simulink model "SPENCER_IK"  (R2023a)
settings: Solver=VariableStepAuto  StartTime=0.0  StopTime=10.0  RelTol=1e-3
model workspace (MAT data in the model file):
  C0 = [0.5 0.25 1]
  P = [1.14564392374 1.14333737187 1.13642700394 1.12494064556 1.10892454825 1.08844320316 1.06357908145 1.03443230217 1.0011202291 0.963776998212 0.922552977508 0.877614161573 ... (300 elements, 100x3)]
  P1 = [0 0 0]
  P5 = [1 0.5 2]
  P6 = [2 2 3]
  P8 = [0 0 1]
  R = 1.14564392374
  X = [0 0.0231772421242 0.0460988496987 0.0685120077079 0.0901695091058 0.110832481399 0.130273021303 0.148276708411 0.164644970158 0.179197271982 0.191773108544 0.202233774026 ... (300 elements, 300x1)]
  Y = [-0.220995 -0.219776262304 -0.216133491346 -0.210106865249 -0.201762854987 -0.191193491238 -0.178515349328 -0.163868263455 -0.147413784385 -0.129333397617 -0.109826521681 -0.0891083086369 ... (300 elements, 300x1)]
  Z = [0 0.00332775919732 0.00665551839465 0.00998327759197 0.0133110367893 0.0166387959866 0.0199665551839 0.0232943143813 0.0266220735786 0.0299498327759 0.0332775919732 0.0366053511706 ... (300 elements, 300x1)]
  a = 0.029995
  alpha = [0; 0.0634665182543; 0.126933036509; 0.190399554763; 0.253866073017; 0.317332591272; 0.380799109526; 0.44426562778; 0.507732146035; 0.571198664289; 0.634665182543; 0.698131700798; 0.761598219052; 0.825064737306; 0.888531255561; 0.951997773815; 1.01546429207; 1.07893081032; 1.14239732858; 1.20586384683; 1.26933036509; 1.33279688334; 1.3962634016; 1.45972991985; 1.5231964381; 1.58666295636; 1.65012947461; 1.71359599287; 1.77706251112; 1.84052902938; 1.90399554763; 1.96746206588; 2.03092858414; 2.09439510239; 2.15786162065; 2.2213281389; 2.28479465716; 2.34826117541; 2.41172769366; 2.47519421192; 2.53866073017; 2.60212724843; 2.66559376668; 2.72906028494; 2.79252680319; 2.85599332145; 2.9194598397; 2.98292635795; 3.04639287621; 3.10985939446; 3.17332591272; 3.23679243097; 3.30025894923; 3.36372546748; 3.42719198573; 3.49065850399; 3.55412502224; 3.6175915405; 3.68105805875; 3.74452457701; 3.80799109526; 3.87145761351; 3.93492413177; 3.99839065002; 4.06185716828; 4.12532368653; 4.18879020479; 4.25225672304; 4.3157232413; 4.37918975955; 4.4426562778; 4.50612279606; 4.56958931431; 4.63305583257; 4.69652235082; 4.75998886908; 4.82345538733; 4.88692190558; 4.95038842384; 5.01385494209; 5.07732146035; 5.1407879786; 5.20425449686; 5.26772101511; 5.33118753336; 5.39465405162; 5.45812056987; 5.52158708813; 5.58505360638; 5.64852012464; 5.71198664289; 5.77545316114; 5.8389196794; 5.90238619765; 5.96585271591; 6.02931923416; 6.09278575242; 6.15625227067; 6.21971878893; 6.28318530718]
  b = 0.191
  del = 0.16432586948
  dp = [-6 3]
  h : matlab.ui.Figure (value not decoded)
  n = 5
  nPt = 100
  nturns = 3
  out = Simulink.SimulationOutput
  out.Data.tout = [0 4.01901829042e-10 2.41141097425e-09 1.24589567003e-08 6.26966853305e-08 3.13885328481e-07 1.56982854424e-06 7.84954462301e-06 3.92481250169e-05 0.000196241026986 0.00063098304072 0.00113846260576 ... (4325 elements, 4325x1)]
  out.Metadata = Simulink.SimulationMetadata
  out.Metadata.ModelInfo.ModelName = 'Spencer_Control_System'
  out.Metadata.ModelInfo.ModelVersion = '1.8'
  out.Metadata.ModelInfo.ModelFilePath = 'C:\Users\Memoh\Desktop\E-Just\Years\Fourth Year\Second Semester\Selected Topics\Projects\Mini-Project_1 Cartesian Robot (SPENCER)\Control System\XML\Spencer_Control_System.slx'
  out.Metadata.ModelInfo.UserID = 'Memoh'
  out.Metadata.ModelInfo.MachineName = 'DESKTOP-OME5LRJ'
  out.Metadata.ModelInfo.Platform = 'PCWIN64'
  out.Metadata.ModelInfo.ModelStructuralChecksum = [3684058528; 2352936037; 269108338; 68946655]
  out.Metadata.ModelInfo.SimulationMode = 'normal'
  out.Metadata.ModelInfo.StartTime = 0
  out.Metadata.ModelInfo.StopTime = 10
  out.Metadata.ModelInfo.SolverInfo.Type = 'Variable-Step'
  out.Metadata.ModelInfo.SolverInfo.Solver = 'ode45'
  out.Metadata.ModelInfo.SolverInfo.MaxStepSize = 0.2
  out.Metadata.ModelInfo.SimulinkVersion.Name = 'Simulink'
  out.Metadata.ModelInfo.SimulinkVersion.Version = '10.7'
  out.Metadata.ModelInfo.SimulinkVersion.Release = '(R2023a)'
  out.Metadata.ModelInfo.SimulinkVersion.Date = '19-Nov-2022'
  out.Metadata.ModelInfo.LoggingInfo.LoggingToFile = 'off'
  out.Metadata.TimingInfo.WallClockTimestampStart = '2023-05-20 02:03:08'
  out.Metadata.TimingInfo.WallClockTimestampStop = '2023-05-20 02:03:21'
  out.Metadata.TimingInfo.InitializationElapsedWallTime = 4.9317965
  out.Metadata.TimingInfo.ExecutionElapsedWallTime = 8.2226035
  out.Metadata.TimingInfo.TerminationElapsedWallTime = 0.0204958
  out.Metadata.TimingInfo.TotalElapsedWallTime = 13.1748958
  out.Metadata.TimingInfo.ProfilerData = 'Profiler is not enabled'
  out.Metadata.ExecutionInfo.StopEvent = 'ReachedStopTime'
  out.Metadata.ExecutionInfo.StopEventSource = []
  out.Metadata.ExecutionInfo.StopEventDescription = 'Reached stop time of 10'
  out.Metadata.ExecutionInfo.ErrorDiagnostic = []
  out.Metadata.ExecutionInfo.WarningDiagnostics.Diagnostic = MSLDiagnostic
  out.Metadata.ExecutionInfo.WarningDiagnostics.Diagnostic.identifier = 'Simulink:Engine:WarnAlgLoopsFound'
  out.Metadata.ExecutionInfo.WarningDiagnostics.Diagnostic.message = 'Block diagram ''<a href="matlab:open_system (''Spencer_Control_System'')">Spencer_Control_System</a>'' contains 1 algebraic loop(s). To see more details about the loops use the command <a href="matlab:Simulink.BlockDiagram.getAlgebraicLoops(bdroot);">Simulink.BlockDiagram.getAlgebraicLoops(''Spencer_Control_System'') </a> or the command line Simulink debugger by typing <a href="matlab:sldebug(bdroot);">sldebug(''Spencer_Control_System'') </a> in the MATLAB command window. To eliminate this message, set <a href="matlab:configset.internal.open(''Spencer_Control_System'',''AlgebraicLoopMsg'');">Algebraic loop</a> to "none".'
  out.Metadata.ExecutionInfo.WarningDiagnostics.Diagnostic.paths = {'Spencer_Control_System'}
  out.Metadata.ExecutionInfo.WarningDiagnostics.Diagnostic.arguments = {'Spencer_Control_System', 1, 'Spencer_Control_System', 'Spencer_Control_System'}
  out.Metadata.ExecutionInfo.WarningDiagnostics.Diagnostic.stack = struct([])
  out.Metadata.ExecutionInfo.WarningDiagnostics.Diagnostic.priority = 2
  out.Metadata.ExecutionInfo.WarningDiagnostics.SimulationPhase = 'Initialization'
  out.Metadata.ExecutionInfo.WarningDiagnostics.SimulationTime = []
  out.Metadata.AppInfo = struct()
  p = 0.199
  phi = [0 0.00188514410656 0.00377028821313 0.00565543231969 0.00754057642626 0.00942572053282 0.0113108646394 0.013196008746 0.0150811528525 0.0169662969591 0.0188514410656 0.0207365851722 ... (10000 elements, 1x10000)]
  phi0 = 2.67794504459
  pos = [8  4; 2  7]
  r = [0 0.000670887481998 0.001341774964 0.00201266244599 0.00268354992799 0.00335443740999 0.00402532489199 0.00469621237399 0.00536709985599 0.00603798733798 0.00670887481998 0.00737976230198 ... (10000 elements, 1x10000)]
  u = [0 0 0 0 0 0 0 0 0 0 0 0 ... (3000 elements, 300x10)]
  v = [0 0.105069988414 0.210139976829 0.315209965243 0.420279953657 0.525349942072 0.630419930486 0.735489918901 0.840559907315 0.945629895729 1.05069988414 1.15576987256 ... (3000 elements, 300x10)]
  v1 = [-0.5 1 0]
  x = [0 0.0231772421242 0.0460988496987 0.0685120077079 0.0901695091058 0.110832481399 0.130273021303 0.148276708411 0.164644970158 0.179197271982 0.191773108544 0.202233774026 ... (3000 elements, 300x10)]
  x1 = [0.220995 0.220995 0.220995 0.220995 0.220995 0.220995 0.220995 0.220995 0.220995 0.220995 0.220995 0.220995 ... (3000 elements, 300x10)]
  x2 = [0 0 0 0 0 0 0 0 0 0 0 0 ... (3000 elements, 300x10)]
  y = [-0.220995 -0.219776262304 -0.216133491346 -0.210106865249 -0.201762854987 -0.191193491238 -0.178515349328 -0.163868263455 -0.147413784385 -0.129333397617 -0.109826521681 -0.0891083086369 ... (3000 elements, 300x10)]
  z = [0 0.00332775919732 0.00665551839465 0.00998327759197 0.0133110367893 0.0166387959866 0.0199665551839 0.0232943143813 0.0266220735786 0.0299498327759 0.0332775919732 0.0366053511706 ... (3000 elements, 300x10)]
undefined symbols (not defined in the file or in its folder): smiData
libraries: sm_lib x27, nesl_utility x10, slpidlib x4, fl_lib x1
(part 1 of 2)
settings Model: Creator=Memoh  LastModifiedBy=Memoh

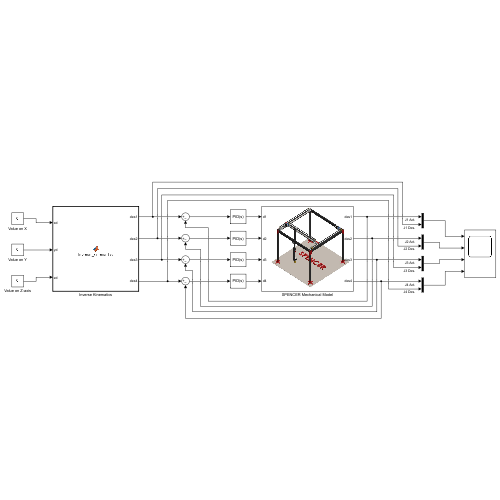
[thumbnail: Simulink's stored preview of the top-level diagram]
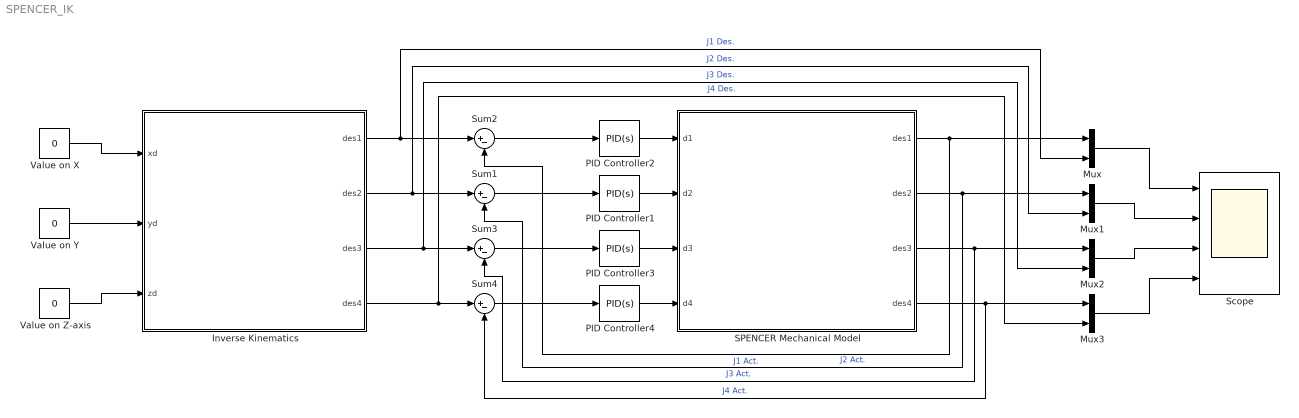
== system SPENCER_IK ==
  Inverse Kinematics : MATLAB Function  TreatAsAtomicUnit=on
  Mux{,1..3} (4 alike) : Mux  Inputs=2
  PID Controller{1..4} (4 alike) : slpidlib/PID Controller  Controller=PID  Form=Parallel  TimeDomain=Continuous-time  UseExternalTs=off  SampleTime=-1  IntegratorMethod=Forward Euler  FilterMethod=Forward Euler  ControllerParametersSource=internal  P=0.03  I=15  UseKiTs=off  D=0  N=100  UseFilter=on  TunerSelectOption=Transfer Function Based (PID Tuner App)  InitialConditionSource=internal  InitialConditionForIntegrator=0  InitialConditionForFilter=0  DifferentiatorICPrevScaledInput=0  ExternalReset=none  TrackingMode=off  Kt=1  LimitOutput=off  SatLimitsSource=internal  UpperSaturationLimit=inf  LowerSaturationLimit=-inf  LinearizeAsGain=on  AntiWindupMode=none  Kb=1  LimitIntegrator=off  UpperIntegratorSaturationLimit=inf  LowerIntegratorSaturationLimit=-inf  POutMin=[]  POutMax=[]  IOutMin=[]  IOutMax=[]  DOutMin=[]  DOutMax=[]  NOutMin=[]  NOutMax=[]  SumOutMin=[]  SumOutMax=[]  SaturationOutMin=[]  SaturationOutMax=[]  PParamMin=[]  PParamMax=[]  IParamMin=[]  IParamMax=[]  DParamMin=[]  DParamMax=[]  NParamMin=[]  NParamMax=[]  KbParamMin=[]  KbParamMax=[]  KtParamMin=[]  KtParamMax=[]  KbOutMin=[]  KbOutMax=[]  KtOutMin=[]  KtOutMax=[]  IntegratorOutMin=[]  IntegratorOutMax=[]  FilterOutMin=[]  FilterOutMax=[]  SumI1OutMin=[]  SumI1OutMax=[]  SumI2OutMin=[]  SumI2OutMax=[]  SumI3OutMin=[]  SumI3OutMax=[]  SumI4OutMin=[]  SumI4OutMax=[]  SumDOutMin=[]  SumDOutMax=[]  DifferentiatorOutMin=[]  DifferentiatorOutMax=[]  FilterDiffOutCoefMin=[]  FilterDiffOutCoefMax=[]  ReciprocalOutMin=[]  ReciprocalOutMax=[]  SumDenOutMin=[]  SumDenOutMax=[]  SumNumOutMin=[]  SumNumOutMax=[]  DivideOutMin=[]  DivideOutMax=[]  UdiffTsProdOutMin=[]  UdiffTsProdOutMax=[]  NTsProdOutMin=[]  NTsProdOutMax=[]  UintegralTsProdOutMin=[]  UintegralTsProdOutMax=[]  UngainTsProdOutMin=[]  UngainTsProdOutMax=[]  ClampingZeroOutDataTypeStr=Inherit: Inherit via back propagation  ClampingZeroOutMin=[]  ClampingZeroOutMax=[]  FilterDenConstantOutDataTypeStr=Inherit: Inherit via back propagation  FilterDenConstantOutMin=[]  FilterDenConstantOutMax=[]  PCopyOutDataTypeStr=Inherit: Inherit via back propagation  PCopyOutMin=[]  PCopyOutMax=[]  NCopyOutDataTypeStr=Inherit: Inherit via back propagation  NCopyOutMin=[]  NCopyOutMax=[]  IntegratorContinuousStateAttributes=''  IntegratorStateMustResolveToSignalObject=off  IntegratorRTWStateStorageClass=Auto  FilterContinuousStateAttributes=''  FilterStateMustResolveToSignalObject=off  FilterRTWStateStorageClass=Auto  ParallelPVariant=InternalParameters  IdealPVariant=Disabled  IVariant=InternalParameters  DVariant=InternalParameters  IntegratorVariant=Continuous  SatVariant=Disabled  AWVariant=Passthrough  PCopyVariant=Disabled  TRVariant=Disabled  FdbkBlocksVariant=Forward  IdealPFdbkVariant=Disabled  SatFdbkVariant=Disabled  DerivativeFilterVariant=ContFilter  NVariant=InternalParameters  NCopyVariant=Disabled  FilterICVariant=InternalICsFilter  IntegratorICVariant=InternalICs  ExternalResetVariant=Disabled  TRSumVariant=Passthrough  SumFdbkVariant=Disabled  SumVariant=Sum_PID  TsampFilterVariant=InternalTs  TsampNgainVariant=Passthrough  TsampIntegralVariant=Disabled_SignalSpec  ExternalSaturationOutDataTypeStr=Inherit: Same as second input
  SPENCER Mechanical Model : Subsystem
      mask Display: image('$imagefile'); % Use "Edit Image" on toolstrip to change.
  Scope : Scope  NumInputPorts=4
  Sum{1..4} (4 alike) : Sum  Inputs=|+-
  Value on X : Constant  Value=0
  Value on Y : Constant  Value=0
  Value on Z-axis : Constant  Value=0
  wires:
  Sum1/1 -> PID Controller1/1
  Sum3/1 -> PID Controller3/1
  Value on Z-axis/1 -> Inverse Kinematics/3(zd)
  Value on Y/1 -> Inverse Kinematics/2(yd)
  Inverse Kinematics/4(des4) -> Sum4/1, Mux3/2  "J4 Des."
  Mux1/1 -> Scope/2
  Value on X/1 -> Inverse Kinematics/1(xd)
  PID Controller3/1 -> SPENCER Mechanical Model/3(d3)
  PID Controller2/1 -> SPENCER Mechanical Model/1(d1)
  PID Controller1/1 -> SPENCER Mechanical Model/2(d2)
  Inverse Kinematics/1(des1) -> Sum2/1, Mux/2  "J1 Des."
  Inverse Kinematics/2(des2) -> Sum1/1, Mux1/2  "J2 Des."
  Mux/1 -> Scope/1
  SPENCER Mechanical Model/1(des1) -> Sum2/2, Mux/1  "J1 Act."
  Mux3/1 -> Scope/4
  SPENCER Mechanical Model/3(des3) -> Sum3/2, Mux2/1  "J3 Act."
  Sum4/1 -> PID Controller4/1
  SPENCER Mechanical Model/2(des2) -> Mux1/1, Sum1/2  "J2 Act."
  Inverse Kinematics/3(des3) -> Sum3/1, Mux2/2  "J3 Des."
  SPENCER Mechanical Model/4(des4) -> Mux3/1, Sum4/2  "J4 Act."
  Sum2/1 -> PID Controller2/1
  PID Controller4/1 -> SPENCER Mechanical Model/4(d4)
  Mux2/1 -> Scope/3
